simulink library "INT_PthSet_TrqCalc"  (R2016b)
settings: Solver=VariableStepAuto  StartTime=0.0  StopTime=10.0  RelTol=1e-3
settings Model: Creator=xuxingpei  LastModifiedBy=xuxingpei

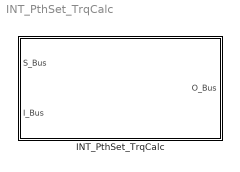
== system INT_PthSet_TrqCalc ==
  INT_PthSet_TrqCalc : Subsystem

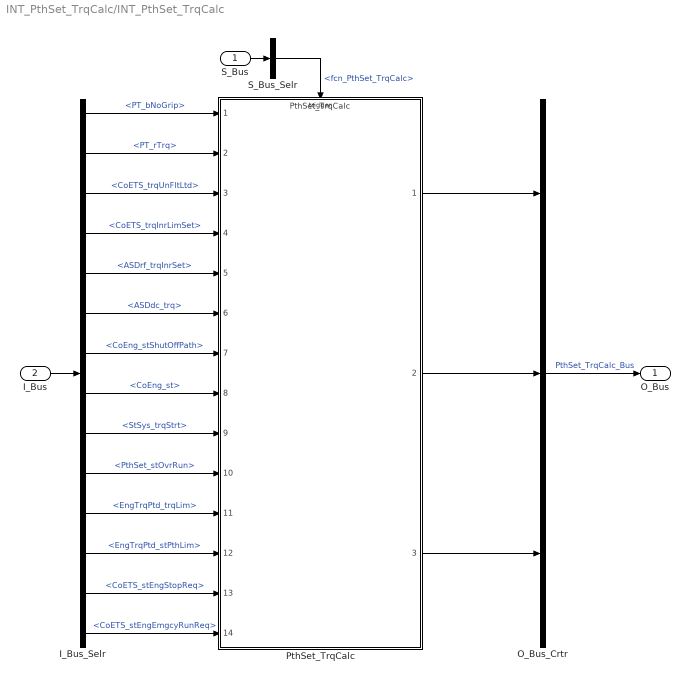
== system INT_PthSet_TrqCalc/INT_PthSet_TrqCalc ==
  S_Bus : Inport
  I_Bus : Inport  Port=2
  I_Bus_Selr : BusSelector  OutputSignals=PT_bNoGrip,PT_rTrq,CoETS_trqUnFltLtd,CoETS_trqInrLimSet,ASDrf_trqInrSet,ASDdc_trq,CoEng_stShutOffPath,CoEng_st,StSys_trqStrt,PthSet_stOvrRun,EngTrqPtd_trqLim,EngTrqPtd_stPthLim,CoETS_stEngStopReq,CoETS_stEngEmgcyRunReq
  O_Bus_Crtr : BusCreator  Inputs=3
  PthSet_TrqCalc : ModelReference  ModelNameDialog=PthSet_TrqCalc  SimulationMode=Normal  ModelReferenceVersion=1.19  TriggerPortName=function  TriggerPortTriggerType=function-call  TriggerPortStatesWhenEnabling=held
  S_Bus_Selr : BusSelector  OutputSignals=fcn_PthSet_TrqCalc
  O_Bus : Outport
  wires:
  S_Bus_Selr/1 -> PthSet_TrqCalc/Trigger  "<fcn_PthSet_TrqCalc>"
  S_Bus/1 -> S_Bus_Selr/1
  I_Bus/1 -> I_Bus_Selr/1
  I_Bus_Selr/1 -> PthSet_TrqCalc/1  "<PT_bNoGrip>"
  I_Bus_Selr/2 -> PthSet_TrqCalc/2  "<PT_rTrq>"
  I_Bus_Selr/3 -> PthSet_TrqCalc/3  "<CoETS_trqUnFltLtd>"
  I_Bus_Selr/4 -> PthSet_TrqCalc/4  "<CoETS_trqInrLimSet>"
  I_Bus_Selr/5 -> PthSet_TrqCalc/5  "<ASDrf_trqInrSet>"
  I_Bus_Selr/6 -> PthSet_TrqCalc/6  "<ASDdc_trq>"
  I_Bus_Selr/7 -> PthSet_TrqCalc/7  "<CoEng_stShutOffPath>"
  I_Bus_Selr/8 -> PthSet_TrqCalc/8  "<CoEng_st>"
  I_Bus_Selr/9 -> PthSet_TrqCalc/9  "<StSys_trqStrt>"
  I_Bus_Selr/10 -> PthSet_TrqCalc/10  "<PthSet_stOvrRun>"
  I_Bus_Selr/11 -> PthSet_TrqCalc/11  "<EngTrqPtd_trqLim>"
  I_Bus_Selr/12 -> PthSet_TrqCalc/12  "<EngTrqPtd_stPthLim>"
  I_Bus_Selr/13 -> PthSet_TrqCalc/13  "<CoETS_stEngStopReq>"
  I_Bus_Selr/14 -> PthSet_TrqCalc/14  "<CoETS_stEngEmgcyRunReq>"
  O_Bus_Crtr/1 -> O_Bus/1  "PthSet_TrqCalc_Bus"
  PthSet_TrqCalc/1 -> O_Bus_Crtr/1
  PthSet_TrqCalc/2 -> O_Bus_Crtr/2
  PthSet_TrqCalc/3 -> O_Bus_Crtr/3
